simulink model "four"  (R2023a)
settings: Solver=FixedStepAuto  StartTime=0.0  StopTime=10  FixedStep=0.01  RelTol=1e-3
settings Model: Creator=evdokiiagalkina  LastModifiedBy=evdokiiagalkina

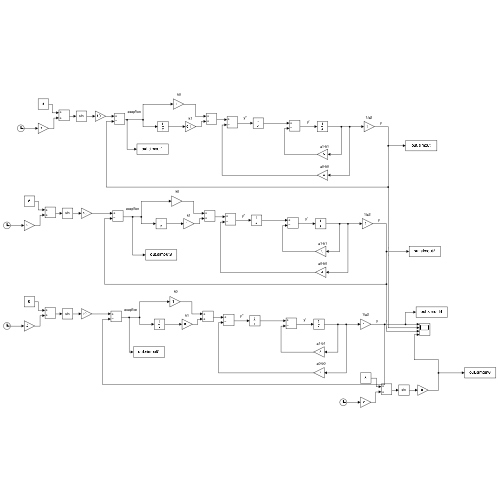
[thumbnail: Simulink's stored preview of the top-level diagram]
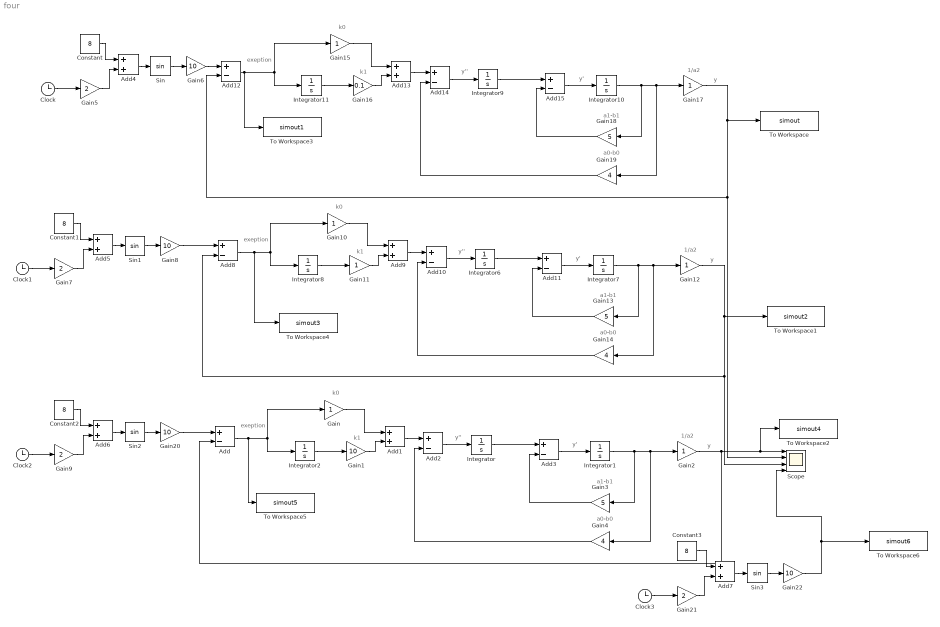
== system four ==
  note: k1
  note: exeption
  note: k0
  note: 1/a2
  note: a0-b0
  note: a1-b1
  note: y
  note: y'
  note: y''
  note: y''
  note: y
  note: exeption
  note: 1/a2
  note: y'
  note: a1-b1
  note: k1
  note: k0
  note: a0-b0
  note: y''
  note: y
  note: exeption
  note: 1/a2
  note: y'
  note: a1-b1
  note: k1
  note: k0
  note: a0-b0
  Add{,2..3,8,10..12,14..15} (9 alike) : Sum  Inputs=+-
  Add{1,4..7,9,13} (7 alike) : Sum
  Clock{,1..3} (4 alike) : Clock
  Constant{,1..3} (4 alike) : Constant  Value=8
  Gain{,2,10..12,15,17} (7 alike) : Gain
  Gain{1,6,8,20,22} (5 alike) : Gain  Gain=10
  Gain13 : Gain  Gain=5
  Gain14 : Gain  Gain=4
  Gain16 : Gain  Gain=0.1
  Gain18 : Gain  Gain=5
  Gain19 : Gain  Gain=4
  Gain{5,7,9,21} (4 alike) : Gain  Gain=2
  Gain3 : Gain  Gain=5
  Gain4 : Gain  Gain=4
  Integrator{,1..2,6..11} (9 alike) : Integrator
  Scope : Scope  NumInputPorts=4
  Sin{,1..3} (4 alike) : Trigonometry
  To Workspace : ToWorkspace  VariableName=simout  SaveFormat=Timeseries  SampleTime=-1
  To Workspace1 : ToWorkspace  VariableName=simout2  SaveFormat=Timeseries  SampleTime=-1
  To Workspace2 : ToWorkspace  VariableName=simout4  SaveFormat=Timeseries  SampleTime=-1
  To Workspace3 : ToWorkspace  VariableName=simout1  SaveFormat=Timeseries  SampleTime=-1
  To Workspace4 : ToWorkspace  VariableName=simout3  SaveFormat=Timeseries  SampleTime=-1
  To Workspace5 : ToWorkspace  VariableName=simout5  SaveFormat=Timeseries  SampleTime=-1
  To Workspace6 : ToWorkspace  VariableName=simout6  SaveFormat=Timeseries  SampleTime=-1
  wires:
  Add/1 -> To Workspace5/1, Gain/1, Integrator2/1
  Integrator/1 -> Add3/1
  Add2/1 -> Integrator/1
  Integrator1/1 -> Gain3/1, Gain4/1, Gain2/1
  Gain2/1 -> To Workspace2/1, Scope/1, Add/2
  Add3/1 -> Integrator1/1
  Gain3/1 -> Add3/2
  Gain4/1 -> Add2/2
  Gain20/1 -> Add/1
  Integrator2/1 -> Gain1/1
  Add1/1 -> Add2/1
  Gain/1 -> Add1/1
  Gain1/1 -> Add1/2
  Gain14/1 -> Add10/2
  Add8/1 -> To Workspace4/1, Gain10/1, Integrator8/1
  Gain12/1 -> Scope/3, Add8/2, To Workspace1/1
  Add10/1 -> Integrator6/1
  Gain10/1 -> Add9/1
  Gain8/1 -> Add8/1
  Gain13/1 -> Add11/2
  Add11/1 -> Integrator7/1
  Integrator7/1 -> Gain13/1, Gain14/1, Gain12/1
  Integrator6/1 -> Add11/1
  Integrator8/1 -> Gain11/1
  Add9/1 -> Add10/1
  Gain11/1 -> Add9/2
  Gain19/1 -> Add14/2
  Add12/1 -> Gain15/1, Integrator11/1, To Workspace3/1
  Gain17/1 -> Scope/2, Add12/2, To Workspace/1
  Add14/1 -> Integrator9/1
  Gain15/1 -> Add13/1
  Gain6/1 -> Add12/1
  Gain18/1 -> Add15/2
  Add15/1 -> Integrator10/1
  Integrator10/1 -> Gain18/1, Gain19/1, Gain17/1
  Integrator9/1 -> Add15/1
  Integrator11/1 -> Gain16/1
  Add13/1 -> Add14/1
  Gain16/1 -> Add13/2
  Gain22/1 -> To Workspace6/1, Scope/4
  Clock/1 -> Gain5/1
  Add4/1 -> Sin/1
  Constant/1 -> Add4/1
  Gain5/1 -> Add4/2
  Sin/1 -> Gain6/1
  Gain7/1 -> Add5/2
  Constant1/1 -> Add5/1
  Add5/1 -> Sin1/1
  Clock1/1 -> Gain7/1
  Sin1/1 -> Gain8/1
  Gain9/1 -> Add6/2
  Constant2/1 -> Add6/1
  Add6/1 -> Sin2/1
  Clock2/1 -> Gain9/1
  Sin2/1 -> Gain20/1
  Gain21/1 -> Add7/2
  Constant3/1 -> Add7/1
  Add7/1 -> Sin3/1
  Clock3/1 -> Gain21/1
  Sin3/1 -> Gain22/1
